simulink model "lab1s"  (R2025a)
settings: Solver=VariableStepAuto  StartTime=0.0  StopTime=10  MaxStep=5e-3  RelTol=1e-3
InitFcn:
  | lambda = 6;
  | gamma = 1;
  | theta = 29 * pi / 180;
settings Model: Creator=zuimio  LastModifiedBy=zuimio

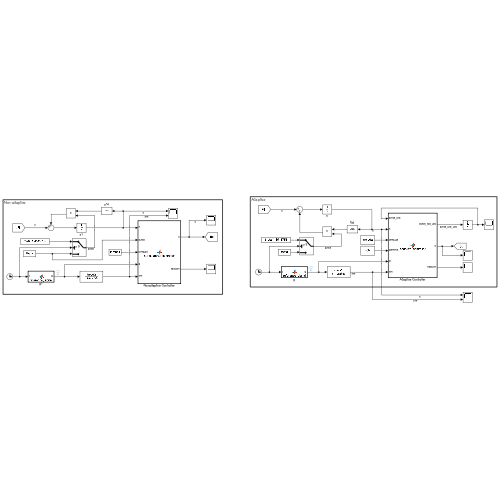
[thumbnail: Simulink's stored preview of the top-level diagram]
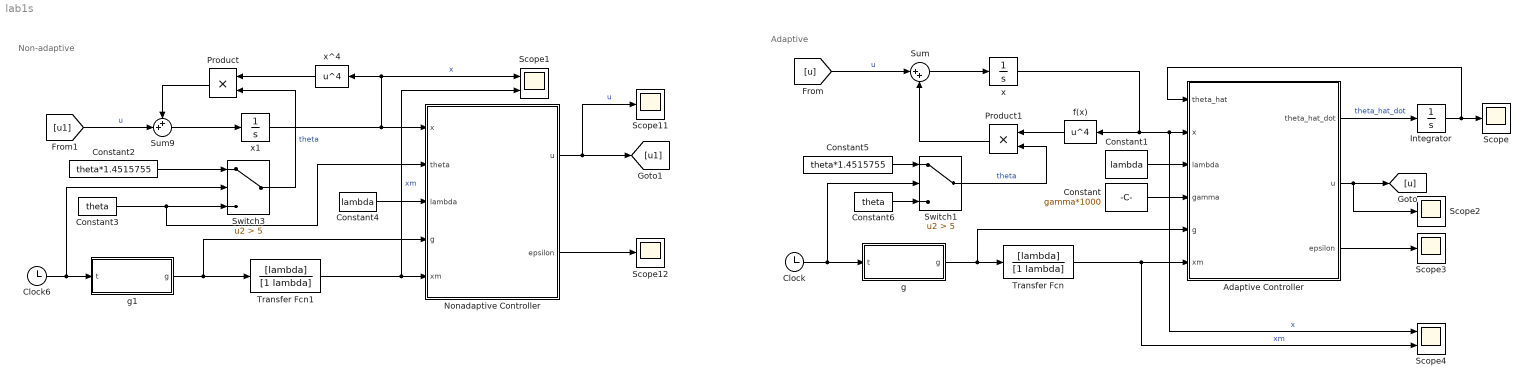
== system lab1s ==
  note: Adaptive
  note: Non-adaptive
  Adaptive Controller : MATLAB Function  TreatAsAtomicUnit=on
  Clock : Clock
  Clock6 : Clock
  Constant : Constant  Value=gamma*1000
  Constant1 : Constant  Value=lambda
  Constant2 : Constant  Value=theta*1.4515755
  Constant3 : Constant  Value=theta
  Constant4 : Constant  Value=lambda
  Constant5 : Constant  Value=theta*1.4515755
  Constant6 : Constant  Value=theta
  Integrator : Integrator
  Nonadaptive Controller : MATLAB Function  TreatAsAtomicUnit=on
  Product : Product
  Product1 : Product
  Scope{,2..3,11..12} (5 alike) : Scope
      Scope settings: ActiveDisplayYMinimum=-0.11489741187399018  ActiveDisplayYMaximum=1.0340767068659118
      Scope11 settings: ActiveDisplayYMinimum=-1  ActiveDisplayYMaximum=1  DataLoggingVariableName=ScopeData11
      Scope12 settings: ActiveDisplayYMinimum=-6.5569891490117023  ActiveDisplayYMaximum=0.72855434989019052  DataLoggingVariableName=ScopeData12
      Scope2 settings: ActiveDisplayYMinimum=-15.101021897347925  ActiveDisplayYMaximum=8.3445579885942127  DataLoggingVariableName=ScopeData2
      Scope3 settings: ActiveDisplayYMinimum=-0.041830356929225987  ActiveDisplayYMaximum=0.027124637570590915  DataLoggingVariableName=ScopeData3
  Scope1 : Scope  NumInputPorts=2
      settings: ActiveDisplayYMinimum=-0.88064968435960678  ActiveDisplayYMaximum=7.9258471592364632
  Scope4 : Scope  NumInputPorts=2
      settings: ActiveDisplayYMinimum=-0.24254711775688406  ActiveDisplayYMaximum=2.182924059811957  DataLoggingVariableName=ScopeData4
  Sum : Sum  Inputs=|++
  Sum9 : Sum  Inputs=++|
  Switch1 : Switch  Criteria=u2 > Threshold  Threshold=5  SaturateOnIntegerOverflow=off  InputSameDT=off
  Switch3 : Switch  Criteria=u2 > Threshold  Threshold=5  SaturateOnIntegerOverflow=off  InputSameDT=off
  Transfer Fcn : TransferFcn  Numerator=[lambda]  Denominator=[1 lambda]
  Transfer Fcn1 : TransferFcn  Numerator=[lambda]  Denominator=[1 lambda]
  f(x) : MATLABFcn  MATLABFcn=u^4
  g : MATLAB Function  TreatAsAtomicUnit=on
  g1 : MATLAB Function  TreatAsAtomicUnit=on
  x : Integrator
  x1 : Integrator
  x^4 : MATLABFcn  MATLABFcn=u^4
  wires:
  x/1 -> Scope4/1, Adaptive Controller/2(x), f(x)/1  "x"
  Sum/1 -> x/1
  [u] -> Sum/1  "u"
  Product1/1 -> Sum/2
  f(x)/1 -> Product1/1
  Integrator/1 -> Scope/1, Adaptive Controller/1(theta_hat)
  Transfer Fcn/1 -> Scope4/2, Adaptive Controller/6(xm)  "xm"
  g/1(g) -> Adaptive Controller/5(g), Transfer Fcn/1
  Constant/1 -> Adaptive Controller/4(gamma)
  Adaptive Controller/1(theta_hat_dot) -> Integrator/1  "theta_hat_dot"
  Constant1/1 -> Adaptive Controller/3(lambda)
  Adaptive Controller/2(u) -> [u], Scope2/1
  Adaptive Controller/3(epsilon) -> Scope3/1
  Nonadaptive Controller/2(epsilon) -> Scope12/1
  Clock6/1 -> g1/1(t), Switch3/2
  Nonadaptive Controller/1(u) -> [u1], Scope11/1  "u"
  g1/1(g) -> Transfer Fcn1/1, Nonadaptive Controller/4(g)
  Transfer Fcn1/1 -> Scope1/2, Nonadaptive Controller/5(xm)  "xm"
  x^4/1 -> Product/1
  Product/1 -> Sum9/1
  [u1] -> Sum9/2  "u"
  Sum9/1 -> x1/1
  x1/1 -> x^4/1, Scope1/1, Nonadaptive Controller/1(x)  "x"
  Constant4/1 -> Nonadaptive Controller/3(lambda)
  Switch3/1 -> Product/2  "theta"
  Constant2/1 -> Switch3/1
  Constant3/1 -> Nonadaptive Controller/2(theta), Switch3/3
  Constant6/1 -> Switch1/3
  Constant5/1 -> Switch1/1
  Switch1/1 -> Product1/2  "theta"
  Clock/1 -> Switch1/2, g/1(t)

== matlab function lab1s/g ==
  data: t input; g output
function g = reference_signal(t)
    g = cos(2*t) .* sin(t) + 1;
end

== matlab function lab1s/Adaptive Controller ==
  data: theta_hat_dot output; theta_hat input; u output; x input; lambda input; gamma input; g input; xm input; epsilon output
function [theta_hat_dot, u, epsilon] = adaptive_controller(theta_hat, x, lambda, gamma, g, xm)

    f_x = x^4;
    
    epsilon = xm - x;
    
    theta_hat_dot = -gamma * f_x * epsilon;

    u = -theta_hat * f_x - lambda * x + lambda * g;
    
end

== matlab function lab1s/Nonadaptive Controller ==
  data: u output; x input; theta input; lambda input; g input; xm input; epsilon output
function [u, epsilon] =nonadaptive_controller(x, theta, lambda, g, xm)

    f_x = x^4;
    
    epsilon = xm - x;

    u = -theta * f_x - lambda * x + lambda * g;
    
end

== matlab function lab1s/g1 ==
  data: t input; g output
function g = reference_signal(t)
    g = cos(2*t) .* sin(t) + 1;
end
